simulink model "pendule_inv_capteur_etu_perso"  (R2023a)
settings: Solver=ode1  StartTime=0.0  StopTime=100  FixedStep=5  RelTol=1e-3
undefined symbols (not defined in the file): g, K, l, x0
settings Model: Creator=ave9761  LastModifiedBy=ave9761
settings SolverCC: ODENIntegrationMethod=ode1

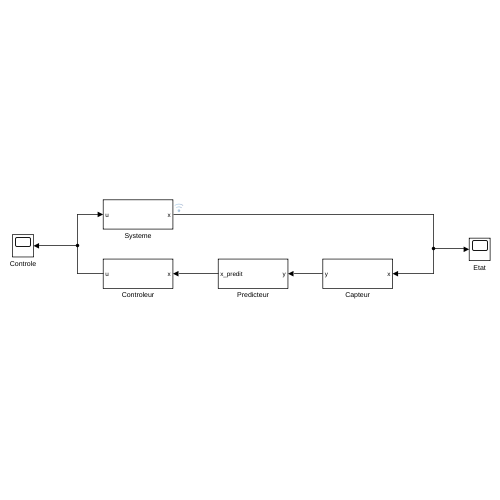
[thumbnail: Simulink's stored preview of the top-level diagram]
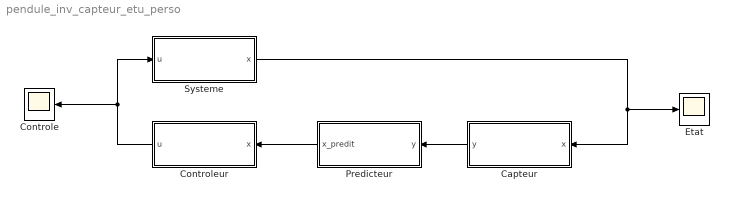
== system pendule_inv_capteur_etu_perso ==
  Capteur : Subsystem
  Controle : Scope
  Controleur : Subsystem
  Etat : Scope
  Predicteur : Subsystem
  Systeme : Subsystem
  wires:
  Controleur/1(u) -> Controle/1, Systeme/1(u)
  Systeme/1(x) -> Capteur/1(x), Etat/1
  Predicteur/1(x_predit) -> Controleur/1(x)
  Capteur/1(y) -> Predicteur/1(y)

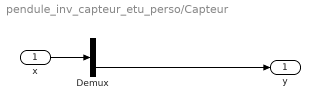
== system pendule_inv_capteur_etu_perso/Capteur ==
  x : Inport
  Demux : Demux  Outputs=2
  y : Outport
  wires:
  x/1 -> Demux/1
  Demux/2 -> y/1

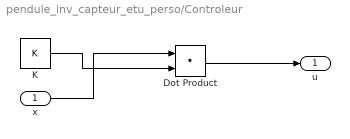
== system pendule_inv_capteur_etu_perso/Controleur ==
  x : Inport
  Dot Product : DotProduct  OutDataTypeStr=Inherit: Inherit via internal rule
  K : Constant  Value=K
  u : Outport
  wires:
  x/1 -> Dot Product/1
  K/1 -> Dot Product/2
  Dot Product/1 -> u/1

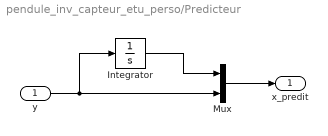
== system pendule_inv_capteur_etu_perso/Predicteur ==
  y : Inport
  Integrator : Integrator  InitialCondition=x0(1)
  Mux : Mux  Inputs=2
  x_predit : Outport
  wires:
  Mux/1 -> x_predit/1
  y/1 -> Integrator/1, Mux/2
  Integrator/1 -> Mux/1

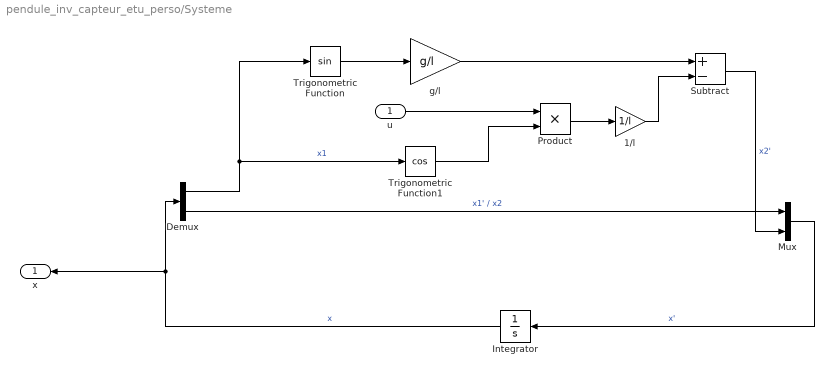
== system pendule_inv_capteur_etu_perso/Systeme ==
  u : Inport
  1/l : Gain  Gain=1/l
  Demux : Demux  Outputs=2
  Integrator : Integrator  InitialCondition=x0
  Mux : Mux  Inputs=2
  Product : Product
  Subtract : Sum  Inputs=+-
  Trigonometric Function : Trigonometry
  Trigonometric Function1 : Trigonometry  Operator=cos
  g/l : Gain  Gain=g/l
  x : Outport
  wires:
  Demux/2 -> Mux/1  "x1' / x2"
  Demux/1 -> Trigonometric Function1/1, Trigonometric Function/1  "x1"
  Trigonometric Function/1 -> g/l/1
  g/l/1 -> Subtract/1
  Subtract/1 -> Mux/2  "x2'"
  u/1 -> Product/1
  1/l/1 -> Subtract/2
  Product/1 -> 1/l/1
  Trigonometric Function1/1 -> Product/2
  Mux/1 -> Integrator/1  "x'"
  Integrator/1 -> x/1, Demux/1  "x"
